simulink model "interp_2"  (Simulink 7.8)
settings: Solver=ode45  StartTime=0.0  StopTime=0.2  RelTol=1e-3
libraries: dspsigops x3, dsparch4 x1
settings Model: Creator=svenhoffmann  LastModifiedBy=josef  ExtModeAutoUpdateStatusClock=off
settings DataIOCC: SignalLoggingName=sigsOut
settings OptimizationCC: InitFltsAndDblsToZero=on
settings DebuggingCC: SaveWithParameterizedLinksMsg=none  SignalResolutionControl=TryResolveAllWithWarning  SolverPrmCheckMsg=none  MultiTaskDSMMsg=warning  MultiTaskCondExecSysMsg=none  FcnCallInpInsideContextMsg=Use local settings  StrictBusMsg=None
settings HardwareCC: TargetUnknown=on
settings RTWCC: IncludeERTFirstTime=on
settings GRTTargetCC: TargetFcnLib=ansi_tfl_tmw.mat

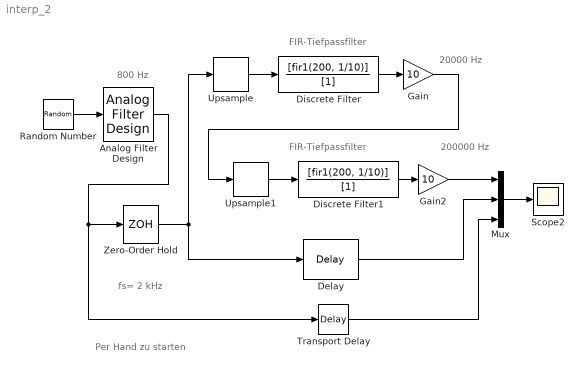
== system interp_2 ==
  note: 800 Hz
  note: fs=
      | 2 kHz
  note: FIR-Tiefpassfilter
  note: FIR-Tiefpassfilter
  note: 20000 Hz
  note: 200000 Hz
  note: Per Hand zu starten
  Analog Filter Design : dsparch4/Analog Filter Design  method=Chebyshev I  filttype=Lowpass  N=8  Wlo=2*pi*800  Whi=80  Rp=2  Rs=40
  Delay : dspsigops/Delay  InputProcessing=Inherited (this choice will be removed - see release notes)  dly_unit=Samples  delay=11  ic_detail=off  dif_ic_for_ch=off  dif_ic_for_dly=off  ic=0  reset_popup=None
  Discrete Filter : DiscreteFilter  Numerator=[fir1(200, 1/10)]  Denominator=[1]
  Discrete Filter1 : DiscreteFilter  Numerator=[fir1(200, 1/10)]  Denominator=[1]
  Gain : Gain  Gain=10  SaturateOnIntegerOverflow=on  OutDataTypeStr=Inherit: Same as input  ParamDataTypeStr=Inherit: Same as input
  Gain2 : Gain  Gain=10  SaturateOnIntegerOverflow=on  OutDataTypeStr=Inherit: Same as input  ParamDataTypeStr=Inherit: Same as input
  Mux : Mux  Inputs=3
  Random Number : RandomNumber  SampleTime=0
  Scope2 : Scope
      settings: TimeRange=0.00974452554744526  YMin=-0.25  YMax=0.15
  Transport Delay : TransportDelay  DelayTime=11/2000
  Upsample : dspsigops/Upsample  N=10  phase=0  InputProcessing=Inherited (this choice will be removed - see release notes)  RateOptions=Allow multirate processing  ic=0  mode=Unused parameter value
  Upsample1 : dspsigops/Upsample  N=10  phase=0  InputProcessing=Inherited (this choice will be removed - see release notes)  RateOptions=Allow multirate processing  ic=0  mode=Unused parameter value
  Zero-Order Hold : ZeroOrderHold  SampleTime=1/2000
  wires:
  Zero-Order Hold/1 -> Upsample/1, Delay/1
  Discrete Filter/1 -> Gain/1
  Upsample/1 -> Discrete Filter/1
  Delay/1 -> Mux/2
  Random Number/1 -> Analog Filter Design/1
  Analog Filter Design/1 -> Zero-Order Hold/1, Transport Delay/1
  Transport Delay/1 -> Mux/3
  Mux/1 -> Scope2/1
  Discrete Filter1/1 -> Gain2/1
  Upsample1/1 -> Discrete Filter1/1
  Gain2/1 -> Mux/1
  Gain/1 -> Upsample1/1
